simulink model "eeg_preview"  (R2013b)
settings: Solver=ode45  StartTime=0.0  StopTime=inf  RelTol=1e-3
undefined symbols (not defined in the file or in its folder): currentCFG_eeg1_UB, UB
libraries: gtecHighspeedLib x2, gUSBamplib x1
settings Model: Creator=geyer_adm  LastModifiedBy=geyer_adm
settings DataIOCC: SignalLoggingSaveFormat=ModelDataLogs
settings DebuggingCC: MultiTaskDSMMsg=warning  MultiTaskCondExecSysMsg=none  StrictBusMsg=None
settings RTWCC: IncludeERTFirstTime=on
settings GRTTargetCC: CodeReplacementLibrary=None  CPPClassGenCompliant=on

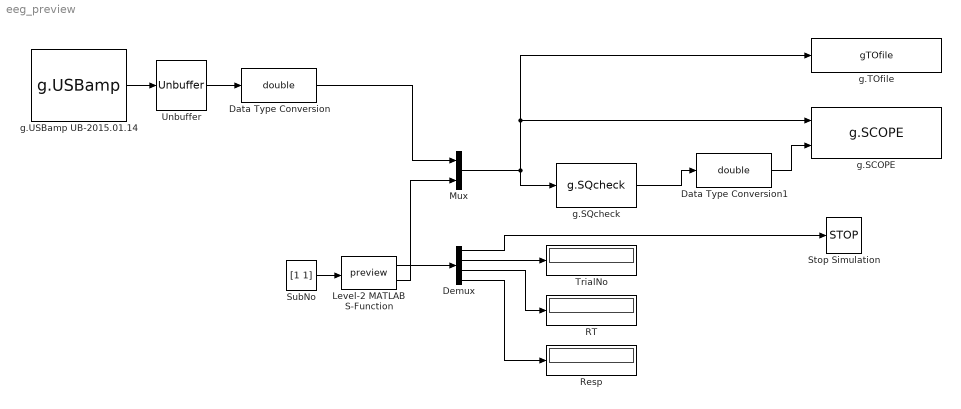
== system eeg_preview ==
  Data Type Conversion : DataTypeConversion  OutDataTypeStr=double
  Data Type Conversion1 : DataTypeConversion  OutDataTypeStr=double
  Demux : Demux
  Level-2 MATLAB S-Function : M-S-Function  FunctionName=preview
  Mux : Mux  Inputs=2
  RT : Display
  Resp : Display
  Stop Simulation : Stop
  SubNo : Constant  Value=[1 1]
  TrialNo : Display
  Unbuffer : Unbuffer  SampleBasedProcessing=Same as frame based
  g.SCOPE : gtecHighspeedLib/g.SCOPE
  g.SQcheck : gtecHighspeedLib/g.SQcheck  updateTime=1000
  g.TOfile : S-Function  FunctionName=gTOfile  Parameters=filename, varname, filesize, blocksize  EnableBusSupport=off  mask(g.TOfile){filename=eeg, varname=y, filesize=500, blocksize=1024}
      mask prompts: varname "Variable:"; filesize "File size [MB]:"; blocksize "Block size [kB]:"
      mask help:
      | The g.TOfile block saves data as a variable into a file. If you have a very large dataset, it will be split into more files, so it is still possible to open it in MATLAB.
      |
      | Parameters:
      | Filename - name of the file, which will be extended with a four digit number
      | Variable - name of the variable, which will be extended with a four digit number
      | File size [MB] - size of the single files in megabytes
      mask Help: web(['file:///' which('gtecHS.htm')],'-helpbrowser');
      mask Callback filename:
      | set_param(gcb, 'LinkStatus', 'none');
      | maskStr = get_param(gcb, 'MaskValues');
      | tmp = sprintf('disp(''%s'')', maskStr{1});
      | set_param(gcb, 'MaskDisplay', tmp);
      | clear maskStr tmp
      mask Callback filesize:
      | maskStr = get_param(gcb, 'MaskValues');
      | mem = memory;
      | maxMem = ((mem.MaxPossibleArrayBytes*0.99)/(1024*1024));
      | if maxMem < str2num(maskStr{3})
      |     errorStr = sprintf('File size too large!\nMaximum file size: %.0f', maxMem);
      |     errordlg(errorStr);
      | end
      | clear maskStr mem maxMem errorStr
      mask Callback blocksize:
      | maskStr = get_param(gcb, 'MaskValues');
      | fileSz = str2num(maskStr{3})*1024;
      | blockSz = str2num(maskStr{4});
      | if fileSz/2 < blockSz
      |     errorStr = sprintf('Block size to large!\nMaximum half of file size');
      |     errorDlg(errorStr);
      | end
      | clear maskStr fileSz blockSz errorStr
      mask Display: disp('eeg')
  g.USBamp UB-2015.01.14 : gUSBamplib/g.USBamp  Priority=2  cfg=currentCFG_eeg1_UB-2015.01.14.cfg  snr=UB-2015.01.14
  wires:
  g.SQcheck/1 -> Data Type Conversion1/1
  Data Type Conversion1/1 -> g.SCOPE/2
  g.USBamp UB-2015.01.14/1 -> Unbuffer/1
  Data Type Conversion/1 -> Mux/1
  Level-2 MATLAB S-Function/2 -> Mux/2
  Mux/1 -> g.SQcheck/1, g.SCOPE/1, g.TOfile/1
  SubNo/1 -> Level-2 MATLAB S-Function/1
  Level-2 MATLAB S-Function/1 -> Demux/1
  Demux/4 -> Resp/1
  Demux/3 -> RT/1
  Demux/2 -> TrialNo/1
  Demux/1 -> Stop Simulation/1
  Unbuffer/1 -> Data Type Conversion/1
